simulink model "ExoskeletonControlModel"  (R2022b)
settings: Solver=ode3  StartTime=0.0  StopTime=inf  FixedStep=Ts  RelTol=1e-3
PreLoadFcn:
  | Ts_IO204 = 0.001;
  | 
  | if ~exist('Ts', 'var')
  | Ts = 0.001;
  | end
  | if ~exist('FPGA_Frequency', 'var')
  | FPGA_Frequency = 75000000;
  | end
  | 
  | ts_IO612 = 1e-3;
  | 
  | load('TargetReached.mat')
  | load('ActualPos_inc.mat')
model workspace (MAT data in the model file):
  DeltaData : timeseries (value not decoded)
  EC45_deg2incs = 2276
  EC60_deg2inc = 5461
  EC90_deg2incs = 7111
  Enc2rad_18bit = 2.3968e-05
  Enc2rad_19bit = 1.1984e-05
  Enc2rad_20bit = 5.9921e-06
  GiulioModel : robotics.RigidBodyTree (value not decoded)
  Giulio_Spheric_model : robotics.RigidBodyTree (value not decoded)
  Offset1_ticks = 571315
  Offset2_ticks = 590938.9928
  Offset3_ticks = 457912.8279
  Offset4_ticks = 482293.9763
  Offset5_ticks = 598735.9316
  Offset_M1 = 1.12645499896
  Offset_M2 = 4.02728553608
  Offset_M3 = 5.48587511336
  Offset_M4 = 2.03717511516
  Offset_M5 = 4.4996674016
  T1_Nm : object (value not decoded)
  T2_Nm : object (value not decoded)
  TBmodel : robotics.RigidBodyTree (value not decoded)
  Ts = 0.002
  Xg : object (value not decoded)
  Yg : object (value not decoded)
  Zg : object (value not decoded)
  a2 = 0.27
  change_variable = 0
  d1 = [0 0 0 0 0 0 0 0 0 0 0 0 ... (30001 elements, 30001x1)]
  d1_1 = 0.21074
  d2 = [0 0 0 0 0 0 0 0 0 0 0 0 ... (30001 elements, 30001x1)]
  d2_1 = 0.04864
  d3 = [0 0 0 0 0 0 0 0 0 0 0 0 ... (30001 elements, 30001x1)]
  d4 = [0 0 0 0 0 0 0 0 0 0 0 0 ... (30001 elements, 30001x1)]
  d5 = [0 0 0 0 0 0 0 0 0 0 0 0 ... (30001 elements, 30001x1)]
  d6 = [0 0 0 0 0 0 0 0 0 0 0 0 ... (30001 elements, 30001x1)]
  ee_x = -0.2852
  ee_y = -0.3683
  ee_z = -0.0386
  enc2rad_EC45 = 7.6699e-06
  enc2rad_EC90 = 2.3969e-05
  k1_Nm_ticks = 0.00923
  k2_Nm_ticks = 0.0257
  k3_Nm_ticks = 0.00692
  k4_Nm_ticks = 0.00729
  k5_Nm_ticks = 0.00641
  lower_lim_m1 = -330000
  lower_lim_m2 = -235302
  lower_lim_m3 = -132865
  lower_lim_m4 = -152732
  lower_lim_m5 = -138363
  lower_lim_m6 = -200325
  m1 = 2.441408578
  m2 = 3.750007
  m3 = 1.56250298
  m4 = 1.56250298
  m5 = 1.56250298
  m6 = 1.56250298
  n_oversampling = 8
  offset_sea_1 = 0.5547
  offset_sea_2 = 2.8595
  offset_sea_3 = 3.5058
  offset_sea_4 = 2.8586
  offset_sea_5 = 2.8736
  params : AKSIM (value not decoded)
  pos_th_neg = -180000
  pos_th_pos = 180000
  q1 = -1819347
  q2 = -196752
  q3 = -596465
  q4 = -556807
  q5 = -573932
  q6 = -489063
  sine = [0 0.187999937334 0.751998997352 1.69199492401 3.0079839574 4.6999608335 6.76791878442 9.21184953835 12.0317433196 15.2275888485 18.7993733417 22.7470825122 ... (12501 elements, 12501x1)]
  start : object (value not decoded)
  switch_admittance = 1
  t1 : object (value not decoded)
  t2 : object (value not decoded)
  torsionalStiffnes_M1 = 384.88
  torsionalStiffnes_M2 = 1500
  torsionalStiffnes_M3 = 901.97
  torsionalStiffnes_M4 = 950.86
  torsionalStiffnes_M5 = 930
  torsionalStiffnes_M6 = 914
  upper_lim_m1 = 340000
  upper_lim_m2 = 95467
  upper_lim_m3 = 164951
  upper_lim_m4 = 210607
  upper_lim_m5 = 252595
  upper_lim_m6 = 96694
  vel_th_neg = -100
  vel_th_pos = 100
  x = 0
undefined symbols (not defined in the file): C, DiscIntNeverNeededParam
libraries: canmsglib x285, speedgoatlib_IO614 x245, simulink x26, slrealtimeloglib x9, simulink_extras x6, robotmaniplib x6
(part 7 of 13)

== system ExoskeletonControlModel/DataProcessing/Working_Chart/GoHome.GoHome_M2.ST1_set_PPM_M2/receive_PDO2_m1 ==
  mode : Inport
  Bus Selector : BusSelector  OutputSignals=mode_m1,interpolation_period_m1
  CAN Write : speedgoatlib_IO614/CAN/CAN Write  id=1  sampleTime=-1  portSelection=3  messageType=CAN  enaStatusPort=off  protl=IO614  ptIdx=2  isFDMod=0
  set_mode : canmsglib/CAN Pack  MsgList=(none)  MsgName=CAN Msg  MsgIDType=Standard (11-bit identifier)  MsgIdentifier=hex2dec('302')  MsgLength=2  Remote=off  ApplyMinMax=off  BusOutput=off  SignalInfo={ 'mode', '0', '8', 'LE', 'unsigned', 'Standard', '0', '1', '0', '-Inf', 'Inf'; 'interpolation time period', '8', '8', 'LE', 'unsigned', 'Standard', '0', '1', '0', '-Inf', 'Inf' }
      settings: DataFormat=manually specified signals
  wires:
  set_mode/1 -> CAN Write/1
  mode/1 -> Bus Selector/1
  Bus Selector/1 -> set_mode/1  "<mode_m1>"
  Bus Selector/2 -> set_mode/2  "<interpolation_period_m1>"

== system ExoskeletonControlModel/DataProcessing/Working_Chart/GoHome.GoHome_M2.ST2_Switch_on_Enable_M2/receive_PDO1_m1 ==
  controlword : Inport
  CAN Write : speedgoatlib_IO614/CAN/CAN Write  id=1  sampleTime=-1  portSelection=3  messageType=CAN  enaStatusPort=off  protl=IO614  ptIdx=2  isFDMod=0
  set_controlword : canmsglib/CAN Pack  MsgList=(none)  MsgName=CAN Msg  MsgIDType=Standard (11-bit identifier)  MsgIdentifier=hex2dec('202')  MsgLength=2  Remote=off  ApplyMinMax=off  BusOutput=off  SignalInfo={ 'controlword', '0', '16', 'LE', 'unsigned', 'Standard', '0', '1', '0', '-Inf', 'Inf' }
      settings: DataFormat=manually specified signals
  wires:
  controlword/1 -> set_controlword/1
  set_controlword/1 -> CAN Write/1

== system ExoskeletonControlModel/DataProcessing/Working_Chart/GoHome.GoHome_M2.ST3_send_target_pos_M2/receive_PDO3_m1 ==
  target_pos : Inport
  CAN Write : speedgoatlib_IO614/CAN/CAN Write  id=1  sampleTime=-1  portSelection=3  messageType=CAN  enaStatusPort=off  protl=IO614  ptIdx=2  isFDMod=0
  set_position : canmsglib/CAN Pack  MsgList=(none)  MsgName=CAN Msg  MsgIDType=Standard (11-bit identifier)  MsgIdentifier=hex2dec('402')  MsgLength=4  Remote=off  ApplyMinMax=off  BusOutput=off  SignalInfo={ 'target position', '0', '32', 'LE', 'signed', 'Standard', '0', '1', '0', '-Inf', 'Inf' }
      settings: DataFormat=manually specified signals
  wires:
  target_pos/1 -> set_position/1
  set_position/1 -> CAN Write/1

== system ExoskeletonControlModel/DataProcessing/Working_Chart/GoHome.GoHome_M2.ST4_Abs_ref_start_immediatly_M2/receive_PDO1_m1 ==
  controlword : Inport
  CAN Write : speedgoatlib_IO614/CAN/CAN Write  id=1  sampleTime=-1  portSelection=3  messageType=CAN  enaStatusPort=off  protl=IO614  ptIdx=2  isFDMod=0
  set_controlword : canmsglib/CAN Pack  MsgList=(none)  MsgName=CAN Msg  MsgIDType=Standard (11-bit identifier)  MsgIdentifier=hex2dec('202')  MsgLength=2  Remote=off  ApplyMinMax=off  BusOutput=off  SignalInfo={ 'controlword', '0', '16', 'LE', 'unsigned', 'Standard', '0', '1', '0', '-Inf', 'Inf' }
      settings: DataFormat=manually specified signals
  wires:
  controlword/1 -> set_controlword/1
  set_controlword/1 -> CAN Write/1

== system ExoskeletonControlModel/DataProcessing/Working_Chart/GoHome.GoHome_M3.ST1_set_PPM_M3/receive_PDO2_m1 ==
  mode : Inport
  Bus Selector : BusSelector  OutputSignals=mode_m1,interpolation_period_m1
  CAN Write : speedgoatlib_IO614/CAN/CAN Write  id=1  sampleTime=-1  portSelection=4  messageType=CAN  enaStatusPort=off  protl=IO614  ptIdx=3  isFDMod=0
  set_mode : canmsglib/CAN Pack  MsgList=(none)  MsgName=CAN Msg  MsgIDType=Standard (11-bit identifier)  MsgIdentifier=hex2dec('301')  MsgLength=2  Remote=off  ApplyMinMax=off  BusOutput=off  SignalInfo={ 'mode', '0', '8', 'LE', 'unsigned', 'Standard', '0', '1', '0', '-Inf', 'Inf'; 'interpolation time period', '8', '8', 'LE', 'unsigned', 'Standard', '0', '1', '0', '-Inf', 'Inf' }
      settings: DataFormat=manually specified signals
  wires:
  set_mode/1 -> CAN Write/1
  mode/1 -> Bus Selector/1
  Bus Selector/1 -> set_mode/1  "<mode_m1>"
  Bus Selector/2 -> set_mode/2  "<interpolation_period_m1>"

== system ExoskeletonControlModel/DataProcessing/Working_Chart/GoHome.GoHome_M3.ST2_Switch_on_Enable_M3/receive_PDO1_m1 ==
  controlword : Inport
  CAN Write : speedgoatlib_IO614/CAN/CAN Write  id=1  sampleTime=-1  portSelection=4  messageType=CAN  enaStatusPort=off  protl=IO614  ptIdx=3  isFDMod=0
  set_controlword : canmsglib/CAN Pack  MsgList=(none)  MsgName=CAN Msg  MsgIDType=Standard (11-bit identifier)  MsgIdentifier=hex2dec('201')  MsgLength=2  Remote=off  ApplyMinMax=off  BusOutput=off  SignalInfo={ 'controlword', '0', '16', 'LE', 'unsigned', 'Standard', '0', '1', '0', '-Inf', 'Inf' }
      settings: DataFormat=manually specified signals
  wires:
  controlword/1 -> set_controlword/1
  set_controlword/1 -> CAN Write/1

== system ExoskeletonControlModel/DataProcessing/Working_Chart/GoHome.GoHome_M3.ST3_send_target_pos_M3/receive_PDO3_m1 ==
  target_pos : Inport
  CAN Write : speedgoatlib_IO614/CAN/CAN Write  id=1  sampleTime=-1  portSelection=4  messageType=CAN  enaStatusPort=off  protl=IO614  ptIdx=3  isFDMod=0
  set_position : canmsglib/CAN Pack  MsgList=(none)  MsgName=CAN Msg  MsgIDType=Standard (11-bit identifier)  MsgIdentifier=hex2dec('401')  MsgLength=4  Remote=off  ApplyMinMax=off  BusOutput=off  SignalInfo={ 'target position', '0', '32', 'LE', 'signed', 'Standard', '0', '1', '0', '-Inf', 'Inf' }
      settings: DataFormat=manually specified signals
  wires:
  target_pos/1 -> set_position/1
  set_position/1 -> CAN Write/1

== system ExoskeletonControlModel/DataProcessing/Working_Chart/GoHome.GoHome_M3.ST4_Abs_ref_start_immediatly_M3/receive_PDO1_m1 ==
  controlword : Inport
  CAN Write : speedgoatlib_IO614/CAN/CAN Write  id=1  sampleTime=-1  portSelection=4  messageType=CAN  enaStatusPort=off  protl=IO614  ptIdx=3  isFDMod=0
  set_controlword : canmsglib/CAN Pack  MsgList=(none)  MsgName=CAN Msg  MsgIDType=Standard (11-bit identifier)  MsgIdentifier=hex2dec('201')  MsgLength=2  Remote=off  ApplyMinMax=off  BusOutput=off  SignalInfo={ 'controlword', '0', '16', 'LE', 'unsigned', 'Standard', '0', '1', '0', '-Inf', 'Inf' }
      settings: DataFormat=manually specified signals
  wires:
  controlword/1 -> set_controlword/1
  set_controlword/1 -> CAN Write/1

== system ExoskeletonControlModel/DataProcessing/Working_Chart/GoHome.GoHome_M4.ST1_set_PPM_M4/receive_PDO2_m1 ==
  mode : Inport
  Bus Selector : BusSelector  OutputSignals=mode_m1,interpolation_period_m1
  CAN Write : speedgoatlib_IO614/CAN/CAN Write  id=1  sampleTime=-1  portSelection=4  messageType=CAN  enaStatusPort=off  protl=IO614  ptIdx=3  isFDMod=0
  set_mode : canmsglib/CAN Pack  MsgList=(none)  MsgName=CAN Msg  MsgIDType=Standard (11-bit identifier)  MsgIdentifier=hex2dec('302')  MsgLength=2  Remote=off  ApplyMinMax=off  BusOutput=off  SignalInfo={ 'mode', '0', '8', 'LE', 'unsigned', 'Standard', '0', '1', '0', '-Inf', 'Inf'; 'interpolation time period', '8', '8', 'LE', 'unsigned', 'Standard', '0', '1', '0', '-Inf', 'Inf' }
      settings: DataFormat=manually specified signals
  wires:
  set_mode/1 -> CAN Write/1
  mode/1 -> Bus Selector/1
  Bus Selector/1 -> set_mode/1  "<mode_m1>"
  Bus Selector/2 -> set_mode/2  "<interpolation_period_m1>"

== system ExoskeletonControlModel/DataProcessing/Working_Chart/GoHome.GoHome_M4.ST2_Switch_on_Enable_M4/receive_PDO1_m1 ==
  controlword : Inport
  CAN Write : speedgoatlib_IO614/CAN/CAN Write  id=1  sampleTime=-1  portSelection=4  messageType=CAN  enaStatusPort=off  protl=IO614  ptIdx=3  isFDMod=0
  set_controlword : canmsglib/CAN Pack  MsgList=(none)  MsgName=CAN Msg  MsgIDType=Standard (11-bit identifier)  MsgIdentifier=hex2dec('202')  MsgLength=2  Remote=off  ApplyMinMax=off  BusOutput=off  SignalInfo={ 'controlword', '0', '16', 'LE', 'unsigned', 'Standard', '0', '1', '0', '-Inf', 'Inf' }
      settings: DataFormat=manually specified signals
  wires:
  controlword/1 -> set_controlword/1
  set_controlword/1 -> CAN Write/1

== system ExoskeletonControlModel/DataProcessing/Working_Chart/GoHome.GoHome_M4.ST3_send_target_pos_M4/receive_PDO3_m1 ==
  target_pos : Inport
  CAN Write : speedgoatlib_IO614/CAN/CAN Write  id=1  sampleTime=-1  portSelection=4  messageType=CAN  enaStatusPort=off  protl=IO614  ptIdx=3  isFDMod=0
  set_position : canmsglib/CAN Pack  MsgList=(none)  MsgName=CAN Msg  MsgIDType=Standard (11-bit identifier)  MsgIdentifier=hex2dec('402')  MsgLength=4  Remote=off  ApplyMinMax=off  BusOutput=off  SignalInfo={ 'target position', '0', '32', 'LE', 'signed', 'Standard', '0', '1', '0', '-Inf', 'Inf' }
      settings: DataFormat=manually specified signals
  wires:
  target_pos/1 -> set_position/1
  set_position/1 -> CAN Write/1

== system ExoskeletonControlModel/DataProcessing/Working_Chart/GoHome.GoHome_M4.ST4_Abs_ref_start_immediatly_M4/receive_PDO1_m1 ==
  controlword : Inport
  CAN Write : speedgoatlib_IO614/CAN/CAN Write  id=1  sampleTime=-1  portSelection=4  messageType=CAN  enaStatusPort=off  protl=IO614  ptIdx=3  isFDMod=0
  set_controlword : canmsglib/CAN Pack  MsgList=(none)  MsgName=CAN Msg  MsgIDType=Standard (11-bit identifier)  MsgIdentifier=hex2dec('202')  MsgLength=2  Remote=off  ApplyMinMax=off  BusOutput=off  SignalInfo={ 'controlword', '0', '16', 'LE', 'unsigned', 'Standard', '0', '1', '0', '-Inf', 'Inf' }
      settings: DataFormat=manually specified signals
  wires:
  controlword/1 -> set_controlword/1
  set_controlword/1 -> CAN Write/1

== system ExoskeletonControlModel/DataProcessing/Working_Chart/GoHome.GoHome_M5.ST1_set_PPM_M5/receive_PDO2_m1 ==
  mode : Inport
  Bus Selector : BusSelector  OutputSignals=mode_m1,interpolation_period_m1
  CAN Write : speedgoatlib_IO614/CAN/CAN Write  id=1  sampleTime=-1  portSelection=4  messageType=CAN  enaStatusPort=off  protl=IO614  ptIdx=3  isFDMod=0
  set_mode : canmsglib/CAN Pack  MsgList=(none)  MsgName=CAN Msg  MsgIDType=Standard (11-bit identifier)  MsgIdentifier=hex2dec('303')  MsgLength=2  Remote=off  ApplyMinMax=off  BusOutput=off  SignalInfo={ 'mode', '0', '8', 'LE', 'unsigned', 'Standard', '0', '1', '0', '-Inf', 'Inf'; 'interpolation time period', '8', '8', 'LE', 'unsigned', 'Standard', '0', '1', '0', '-Inf', 'Inf' }
      settings: DataFormat=manually specified signals
  wires:
  set_mode/1 -> CAN Write/1
  mode/1 -> Bus Selector/1
  Bus Selector/1 -> set_mode/1  "<mode_m1>"
  Bus Selector/2 -> set_mode/2  "<interpolation_period_m1>"

== system ExoskeletonControlModel/DataProcessing/Working_Chart/GoHome.GoHome_M5.ST2_Switch_on_Enable_M5/receive_PDO1_m1 ==
  controlword : Inport
  CAN Write : speedgoatlib_IO614/CAN/CAN Write  id=1  sampleTime=-1  portSelection=4  messageType=CAN  enaStatusPort=off  protl=IO614  ptIdx=3  isFDMod=0
  set_controlword : canmsglib/CAN Pack  MsgList=(none)  MsgName=CAN Msg  MsgIDType=Standard (11-bit identifier)  MsgIdentifier=hex2dec('203')  MsgLength=2  Remote=off  ApplyMinMax=off  BusOutput=off  SignalInfo={ 'controlword', '0', '16', 'LE', 'unsigned', 'Standard', '0', '1', '0', '-Inf', 'Inf' }
      settings: DataFormat=manually specified signals
  wires:
  controlword/1 -> set_controlword/1
  set_controlword/1 -> CAN Write/1

== system ExoskeletonControlModel/DataProcessing/Working_Chart/GoHome.GoHome_M5.ST3_send_target_pos_M5/receive_PDO3_m1 ==
  target_pos : Inport
  CAN Write : speedgoatlib_IO614/CAN/CAN Write  id=1  sampleTime=-1  portSelection=4  messageType=CAN  enaStatusPort=off  protl=IO614  ptIdx=3  isFDMod=0
  set_position : canmsglib/CAN Pack  MsgList=(none)  MsgName=CAN Msg  MsgIDType=Standard (11-bit identifier)  MsgIdentifier=hex2dec('403')  MsgLength=4  Remote=off  ApplyMinMax=off  BusOutput=off  SignalInfo={ 'target position', '0', '32', 'LE', 'signed', 'Standard', '0', '1', '0', '-Inf', 'Inf' }
      settings: DataFormat=manually specified signals
  wires:
  target_pos/1 -> set_position/1
  set_position/1 -> CAN Write/1

== system ExoskeletonControlModel/DataProcessing/Working_Chart/GoHome.GoHome_M5.ST4_Abs_ref_start_immediatly_M5/receive_PDO1_m1 ==
  controlword : Inport
  CAN Write : speedgoatlib_IO614/CAN/CAN Write  id=1  sampleTime=-1  portSelection=4  messageType=CAN  enaStatusPort=off  protl=IO614  ptIdx=3  isFDMod=0
  set_controlword : canmsglib/CAN Pack  MsgList=(none)  MsgName=CAN Msg  MsgIDType=Standard (11-bit identifier)  MsgIdentifier=hex2dec('203')  MsgLength=2  Remote=off  ApplyMinMax=off  BusOutput=off  SignalInfo={ 'controlword', '0', '16', 'LE', 'unsigned', 'Standard', '0', '1', '0', '-Inf', 'Inf' }
      settings: DataFormat=manually specified signals
  wires:
  controlword/1 -> set_controlword/1
  set_controlword/1 -> CAN Write/1

== system ExoskeletonControlModel/DataProcessing/Working_Chart/GoHome.GoHome_M6.ST1_set_PPM_M6/receive_PDO2_m1 ==
  mode : Inport
  Bus Selector : BusSelector  OutputSignals=mode_m1,interpolation_period_m1
  CAN Write : speedgoatlib_IO614/CAN/CAN Write  id=1  sampleTime=-1  portSelection=4  messageType=CAN  enaStatusPort=off  protl=IO614  ptIdx=3  isFDMod=0
  set_mode : canmsglib/CAN Pack  MsgList=(none)  MsgName=CAN Msg  MsgIDType=Standard (11-bit identifier)  MsgIdentifier=hex2dec('304')  MsgLength=2  Remote=off  ApplyMinMax=off  BusOutput=off  SignalInfo={ 'mode', '0', '8', 'LE', 'unsigned', 'Standard', '0', '1', '0', '-Inf', 'Inf'; 'interpolation time period', '8', '8', 'LE', 'unsigned', 'Standard', '0', '1', '0', '-Inf', 'Inf' }
      settings: DataFormat=manually specified signals
  wires:
  set_mode/1 -> CAN Write/1
  mode/1 -> Bus Selector/1
  Bus Selector/1 -> set_mode/1  "<mode_m1>"
  Bus Selector/2 -> set_mode/2  "<interpolation_period_m1>"

== system ExoskeletonControlModel/DataProcessing/Working_Chart/GoHome.GoHome_M6.ST2_Switch_on_Enable_M6/receive_PDO1_m1 ==
  controlword : Inport
  CAN Write : speedgoatlib_IO614/CAN/CAN Write  id=1  sampleTime=-1  portSelection=4  messageType=CAN  enaStatusPort=off  protl=IO614  ptIdx=3  isFDMod=0
  set_controlword : canmsglib/CAN Pack  MsgList=(none)  MsgName=CAN Msg  MsgIDType=Standard (11-bit identifier)  MsgIdentifier=hex2dec('204')  MsgLength=2  Remote=off  ApplyMinMax=off  BusOutput=off  SignalInfo={ 'controlword', '0', '16', 'LE', 'unsigned', 'Standard', '0', '1', '0', '-Inf', 'Inf' }
      settings: DataFormat=manually specified signals
  wires:
  controlword/1 -> set_controlword/1
  set_controlword/1 -> CAN Write/1

== system ExoskeletonControlModel/DataProcessing/Working_Chart/GoHome.GoHome_M6.ST3_send_target_pos_M6/receive_PDO3_m1 ==
  target_pos : Inport
  CAN Write : speedgoatlib_IO614/CAN/CAN Write  id=1  sampleTime=-1  portSelection=4  messageType=CAN  enaStatusPort=off  protl=IO614  ptIdx=3  isFDMod=0
  set_position : canmsglib/CAN Pack  MsgList=(none)  MsgName=CAN Msg  MsgIDType=Standard (11-bit identifier)  MsgIdentifier=hex2dec('404')  MsgLength=4  Remote=off  ApplyMinMax=off  BusOutput=off  SignalInfo={ 'target position', '0', '32', 'LE', 'signed', 'Standard', '0', '1', '0', '-Inf', 'Inf' }
      settings: DataFormat=manually specified signals
  wires:
  target_pos/1 -> set_position/1
  set_position/1 -> CAN Write/1

== system ExoskeletonControlModel/DataProcessing/Working_Chart/GoHome.GoHome_M6.ST4_Abs_ref_start_immediatly_M6/receive_PDO1_m1 ==
  controlword : Inport
  CAN Write : speedgoatlib_IO614/CAN/CAN Write  id=1  sampleTime=-1  portSelection=4  messageType=CAN  enaStatusPort=off  protl=IO614  ptIdx=3  isFDMod=0
  set_controlword : canmsglib/CAN Pack  MsgList=(none)  MsgName=CAN Msg  MsgIDType=Standard (11-bit identifier)  MsgIdentifier=hex2dec('204')  MsgLength=2  Remote=off  ApplyMinMax=off  BusOutput=off  SignalInfo={ 'controlword', '0', '16', 'LE', 'unsigned', 'Standard', '0', '1', '0', '-Inf', 'Inf' }
      settings: DataFormat=manually specified signals
  wires:
  controlword/1 -> set_controlword/1
  set_controlword/1 -> CAN Write/1

== system ExoskeletonControlModel/DataProcessing/Working_Chart/Transparency.Block_not_recorded_joints.ST1_set_CSP_M1/receive_PDO2_m1 ==
  mode : Inport
  Bus Selector : BusSelector  OutputSignals=mode_m1,interpolation_period_m1
  CAN Write : speedgoatlib_IO614/CAN/CAN Write  id=1  sampleTime=-1  portSelection=3  messageType=CAN  enaStatusPort=off  protl=IO614  ptIdx=2  isFDMod=0
  set_mode : canmsglib/CAN Pack  MsgList=(none)  MsgName=CAN Msg  MsgIDType=Standard (11-bit identifier)  MsgIdentifier=hex2dec('301')  MsgLength=2  Remote=off  ApplyMinMax=off  BusOutput=off  SignalInfo={ 'mode', '0', '8', 'LE', 'unsigned', 'Standard', '0', '1', '0', '-Inf', 'Inf'; 'interpolation time period', '8', '8', 'LE', 'unsigned', 'Standard', '0', '1', '0', '-Inf', 'Inf' }
      settings: DataFormat=manually specified signals
  wires:
  set_mode/1 -> CAN Write/1
  mode/1 -> Bus Selector/1
  Bus Selector/1 -> set_mode/1  "<mode_m1>"
  Bus Selector/2 -> set_mode/2  "<interpolation_period_m1>"

== system ExoskeletonControlModel/DataProcessing/Working_Chart/Transparency.Block_not_recorded_joints.ST1_set_CSP_M6/receive_PDO2_m1 ==
  mode : Inport
  Bus Selector : BusSelector  OutputSignals=mode_m1,interpolation_period_m1
  CAN Write : speedgoatlib_IO614/CAN/CAN Write  id=1  sampleTime=-1  portSelection=4  messageType=CAN  enaStatusPort=off  protl=IO614  ptIdx=3  isFDMod=0
  set_mode : canmsglib/CAN Pack  MsgList=(none)  MsgName=CAN Msg  MsgIDType=Standard (11-bit identifier)  MsgIdentifier=hex2dec('304')  MsgLength=2  Remote=off  ApplyMinMax=off  BusOutput=off  SignalInfo={ 'mode', '0', '8', 'LE', 'unsigned', 'Standard', '0', '1', '0', '-Inf', 'Inf'; 'interpolation time period', '8', '8', 'LE', 'unsigned', 'Standard', '0', '1', '0', '-Inf', 'Inf' }
      settings: DataFormat=manually specified signals
  wires:
  set_mode/1 -> CAN Write/1
  mode/1 -> Bus Selector/1
  Bus Selector/1 -> set_mode/1  "<mode_m1>"
  Bus Selector/2 -> set_mode/2  "<interpolation_period_m1>"

== system ExoskeletonControlModel/DataProcessing/Working_Chart/Transparency.GoToExerciseHome.GoHome_M1.ST1_set_PPM_M1/receive_PDO2_m1 ==
  mode : Inport
  Bus Selector : BusSelector  OutputSignals=mode_m1,interpolation_period_m1
  CAN Write : speedgoatlib_IO614/CAN/CAN Write  id=1  sampleTime=-1  portSelection=3  messageType=CAN  enaStatusPort=off  protl=IO614  ptIdx=2  isFDMod=0
  set_mode : canmsglib/CAN Pack  MsgList=(none)  MsgName=CAN Msg  MsgIDType=Standard (11-bit identifier)  MsgIdentifier=hex2dec('301')  MsgLength=2  Remote=off  ApplyMinMax=off  BusOutput=off  SignalInfo={ 'mode', '0', '8', 'LE', 'unsigned', 'Standard', '0', '1', '0', '-Inf', 'Inf'; 'interpolation time period', '8', '8', 'LE', 'unsigned', 'Standard', '0', '1', '0', '-Inf', 'Inf' }
      settings: DataFormat=manually specified signals
  wires:
  set_mode/1 -> CAN Write/1
  mode/1 -> Bus Selector/1
  Bus Selector/1 -> set_mode/1  "<mode_m1>"
  Bus Selector/2 -> set_mode/2  "<interpolation_period_m1>"

== system ExoskeletonControlModel/DataProcessing/Working_Chart/Transparency.GoToExerciseHome.GoHome_M1.ST2_Switch_on_Enable_M1/receive_PDO1_m1 ==
  controlword : Inport
  CAN Write : speedgoatlib_IO614/CAN/CAN Write  id=1  sampleTime=-1  portSelection=3  messageType=CAN  enaStatusPort=off  protl=IO614  ptIdx=2  isFDMod=0
  set_controlword : canmsglib/CAN Pack  MsgList=(none)  MsgName=CAN Msg  MsgIDType=Standard (11-bit identifier)  MsgIdentifier=hex2dec('201')  MsgLength=2  Remote=off  ApplyMinMax=off  BusOutput=off  SignalInfo={ 'controlword', '0', '16', 'LE', 'unsigned', 'Standard', '0', '1', '0', '-Inf', 'Inf' }
      settings: DataFormat=manually specified signals
  wires:
  controlword/1 -> set_controlword/1
  set_controlword/1 -> CAN Write/1

== system ExoskeletonControlModel/DataProcessing/Working_Chart/Transparency.GoToExerciseHome.GoHome_M1.ST3_send_target_pos_M1/receive_PDO3_m1 ==
  target_pos : Inport
  CAN Write : speedgoatlib_IO614/CAN/CAN Write  id=1  sampleTime=-1  portSelection=3  messageType=CAN  enaStatusPort=off  protl=IO614  ptIdx=2  isFDMod=0
  set_position : canmsglib/CAN Pack  MsgList=(none)  MsgName=CAN Msg  MsgIDType=Standard (11-bit identifier)  MsgIdentifier=hex2dec('401')  MsgLength=4  Remote=off  ApplyMinMax=off  BusOutput=off  SignalInfo={ 'target position', '0', '32', 'LE', 'signed', 'Standard', '0', '1', '0', '-Inf', 'Inf' }
      settings: DataFormat=manually specified signals
  wires:
  target_pos/1 -> set_position/1
  set_position/1 -> CAN Write/1

== system ExoskeletonControlModel/DataProcessing/Working_Chart/Transparency.GoToExerciseHome.GoHome_M1.ST4_Abs_ref_start_immediatly_M1/receive_PDO1_m1 ==
  controlword : Inport
  CAN Write : speedgoatlib_IO614/CAN/CAN Write  id=1  sampleTime=-1  portSelection=3  messageType=CAN  enaStatusPort=off  protl=IO614  ptIdx=2  isFDMod=0
  set_controlword : canmsglib/CAN Pack  MsgList=(none)  MsgName=CAN Msg  MsgIDType=Standard (11-bit identifier)  MsgIdentifier=hex2dec('201')  MsgLength=2  Remote=off  ApplyMinMax=off  BusOutput=off  SignalInfo={ 'controlword', '0', '16', 'LE', 'unsigned', 'Standard', '0', '1', '0', '-Inf', 'Inf' }
      settings: DataFormat=manually specified signals
  wires:
  controlword/1 -> set_controlword/1
  set_controlword/1 -> CAN Write/1

== system ExoskeletonControlModel/DataProcessing/Working_Chart/Transparency.GoToExerciseHome.GoHome_M2.ST1_set_PPM_M2/receive_PDO2_m1 ==
  mode : Inport
  Bus Selector : BusSelector  OutputSignals=mode_m1,interpolation_period_m1
  CAN Write : speedgoatlib_IO614/CAN/CAN Write  id=1  sampleTime=-1  portSelection=3  messageType=CAN  enaStatusPort=off  protl=IO614  ptIdx=2  isFDMod=0
  set_mode : canmsglib/CAN Pack  MsgList=(none)  MsgName=CAN Msg  MsgIDType=Standard (11-bit identifier)  MsgIdentifier=hex2dec('302')  MsgLength=2  Remote=off  ApplyMinMax=off  BusOutput=off  SignalInfo={ 'mode', '0', '8', 'LE', 'unsigned', 'Standard', '0', '1', '0', '-Inf', 'Inf'; 'interpolation time period', '8', '8', 'LE', 'unsigned', 'Standard', '0', '1', '0', '-Inf', 'Inf' }
      settings: DataFormat=manually specified signals
  wires:
  set_mode/1 -> CAN Write/1
  mode/1 -> Bus Selector/1
  Bus Selector/1 -> set_mode/1  "<mode_m1>"
  Bus Selector/2 -> set_mode/2  "<interpolation_period_m1>"

== system ExoskeletonControlModel/DataProcessing/Working_Chart/Transparency.GoToExerciseHome.GoHome_M2.ST2_Switch_on_Enable_M2/receive_PDO1_m1 ==
  controlword : Inport
  CAN Write : speedgoatlib_IO614/CAN/CAN Write  id=1  sampleTime=-1  portSelection=3  messageType=CAN  enaStatusPort=off  protl=IO614  ptIdx=2  isFDMod=0
  set_controlword : canmsglib/CAN Pack  MsgList=(none)  MsgName=CAN Msg  MsgIDType=Standard (11-bit identifier)  MsgIdentifier=hex2dec('202')  MsgLength=2  Remote=off  ApplyMinMax=off  BusOutput=off  SignalInfo={ 'controlword', '0', '16', 'LE', 'unsigned', 'Standard', '0', '1', '0', '-Inf', 'Inf' }
      settings: DataFormat=manually specified signals
  wires:
  controlword/1 -> set_controlword/1
  set_controlword/1 -> CAN Write/1

== system ExoskeletonControlModel/DataProcessing/Working_Chart/Transparency.GoToExerciseHome.GoHome_M2.ST3_send_target_pos_M2/receive_PDO3_m1 ==
  target_pos : Inport
  CAN Write : speedgoatlib_IO614/CAN/CAN Write  id=1  sampleTime=-1  portSelection=3  messageType=CAN  enaStatusPort=off  protl=IO614  ptIdx=2  isFDMod=0
  set_position : canmsglib/CAN Pack  MsgList=(none)  MsgName=CAN Msg  MsgIDType=Standard (11-bit identifier)  MsgIdentifier=hex2dec('402')  MsgLength=4  Remote=off  ApplyMinMax=off  BusOutput=off  SignalInfo={ 'target position', '0', '32', 'LE', 'signed', 'Standard', '0', '1', '0', '-Inf', 'Inf' }
      settings: DataFormat=manually specified signals
  wires:
  target_pos/1 -> set_position/1
  set_position/1 -> CAN Write/1

== system ExoskeletonControlModel/DataProcessing/Working_Chart/Transparency.GoToExerciseHome.GoHome_M2.ST4_Abs_ref_start_immediatly_M2/receive_PDO1_m1 ==
  controlword : Inport
  CAN Write : speedgoatlib_IO614/CAN/CAN Write  id=1  sampleTime=-1  portSelection=3  messageType=CAN  enaStatusPort=off  protl=IO614  ptIdx=2  isFDMod=0
  set_controlword : canmsglib/CAN Pack  MsgList=(none)  MsgName=CAN Msg  MsgIDType=Standard (11-bit identifier)  MsgIdentifier=hex2dec('202')  MsgLength=2  Remote=off  ApplyMinMax=off  BusOutput=off  SignalInfo={ 'controlword', '0', '16', 'LE', 'unsigned', 'Standard', '0', '1', '0', '-Inf', 'Inf' }
      settings: DataFormat=manually specified signals
  wires:
  controlword/1 -> set_controlword/1
  set_controlword/1 -> CAN Write/1

== system ExoskeletonControlModel/DataProcessing/Working_Chart/Transparency.GoToExerciseHome.GoHome_M3.ST1_set_PPM_M3/receive_PDO2_m1 ==
  mode : Inport
  Bus Selector : BusSelector  OutputSignals=mode_m1,interpolation_period_m1
  CAN Write : speedgoatlib_IO614/CAN/CAN Write  id=1  sampleTime=-1  portSelection=4  messageType=CAN  enaStatusPort=off  protl=IO614  ptIdx=3  isFDMod=0
  set_mode : canmsglib/CAN Pack  MsgList=(none)  MsgName=CAN Msg  MsgIDType=Standard (11-bit identifier)  MsgIdentifier=hex2dec('301')  MsgLength=2  Remote=off  ApplyMinMax=off  BusOutput=off  SignalInfo={ 'mode', '0', '8', 'LE', 'unsigned', 'Standard', '0', '1', '0', '-Inf', 'Inf'; 'interpolation time period', '8', '8', 'LE', 'unsigned', 'Standard', '0', '1', '0', '-Inf', 'Inf' }
      settings: DataFormat=manually specified signals
  wires:
  set_mode/1 -> CAN Write/1
  mode/1 -> Bus Selector/1
  Bus Selector/1 -> set_mode/1  "<mode_m1>"
  Bus Selector/2 -> set_mode/2  "<interpolation_period_m1>"

== system ExoskeletonControlModel/DataProcessing/Working_Chart/Transparency.GoToExerciseHome.GoHome_M3.ST2_Switch_on_Enable_M3/receive_PDO1_m1 ==
  controlword : Inport
  CAN Write : speedgoatlib_IO614/CAN/CAN Write  id=1  sampleTime=-1  portSelection=4  messageType=CAN  enaStatusPort=off  protl=IO614  ptIdx=3  isFDMod=0
  set_controlword : canmsglib/CAN Pack  MsgList=(none)  MsgName=CAN Msg  MsgIDType=Standard (11-bit identifier)  MsgIdentifier=hex2dec('201')  MsgLength=2  Remote=off  ApplyMinMax=off  BusOutput=off  SignalInfo={ 'controlword', '0', '16', 'LE', 'unsigned', 'Standard', '0', '1', '0', '-Inf', 'Inf' }
      settings: DataFormat=manually specified signals
  wires:
  controlword/1 -> set_controlword/1
  set_controlword/1 -> CAN Write/1

== system ExoskeletonControlModel/DataProcessing/Working_Chart/Transparency.GoToExerciseHome.GoHome_M3.ST3_send_target_pos_M3/receive_PDO3_m1 ==
  target_pos : Inport
  CAN Write : speedgoatlib_IO614/CAN/CAN Write  id=1  sampleTime=-1  portSelection=4  messageType=CAN  enaStatusPort=off  protl=IO614  ptIdx=3  isFDMod=0
  set_position : canmsglib/CAN Pack  MsgList=(none)  MsgName=CAN Msg  MsgIDType=Standard (11-bit identifier)  MsgIdentifier=hex2dec('401')  MsgLength=4  Remote=off  ApplyMinMax=off  BusOutput=off  SignalInfo={ 'target position', '0', '32', 'LE', 'signed', 'Standard', '0', '1', '0', '-Inf', 'Inf' }
      settings: DataFormat=manually specified signals
  wires:
  target_pos/1 -> set_position/1
  set_position/1 -> CAN Write/1

== system ExoskeletonControlModel/DataProcessing/Working_Chart/Transparency.GoToExerciseHome.GoHome_M3.ST4_Abs_ref_start_immediatly_M3/receive_PDO1_m1 ==
  controlword : Inport
  CAN Write : speedgoatlib_IO614/CAN/CAN Write  id=1  sampleTime=-1  portSelection=4  messageType=CAN  enaStatusPort=off  protl=IO614  ptIdx=3  isFDMod=0
  set_controlword : canmsglib/CAN Pack  MsgList=(none)  MsgName=CAN Msg  MsgIDType=Standard (11-bit identifier)  MsgIdentifier=hex2dec('201')  MsgLength=2  Remote=off  ApplyMinMax=off  BusOutput=off  SignalInfo={ 'controlword', '0', '16', 'LE', 'unsigned', 'Standard', '0', '1', '0', '-Inf', 'Inf' }
      settings: DataFormat=manually specified signals
  wires:
  controlword/1 -> set_controlword/1
  set_controlword/1 -> CAN Write/1

== system ExoskeletonControlModel/DataProcessing/Working_Chart/Transparency.GoToExerciseHome.GoHome_M4.ST1_set_PPM_M4/receive_PDO2_m1 ==
  mode : Inport
  Bus Selector : BusSelector  OutputSignals=mode_m1,interpolation_period_m1
  CAN Write : speedgoatlib_IO614/CAN/CAN Write  id=1  sampleTime=-1  portSelection=4  messageType=CAN  enaStatusPort=off  protl=IO614  ptIdx=3  isFDMod=0
  set_mode : canmsglib/CAN Pack  MsgList=(none)  MsgName=CAN Msg  MsgIDType=Standard (11-bit identifier)  MsgIdentifier=hex2dec('302')  MsgLength=2  Remote=off  ApplyMinMax=off  BusOutput=off  SignalInfo={ 'mode', '0', '8', 'LE', 'unsigned', 'Standard', '0', '1', '0', '-Inf', 'Inf'; 'interpolation time period', '8', '8', 'LE', 'unsigned', 'Standard', '0', '1', '0', '-Inf', 'Inf' }
      settings: DataFormat=manually specified signals
  wires:
  set_mode/1 -> CAN Write/1
  mode/1 -> Bus Selector/1
  Bus Selector/1 -> set_mode/1  "<mode_m1>"
  Bus Selector/2 -> set_mode/2  "<interpolation_period_m1>"

== system ExoskeletonControlModel/DataProcessing/Working_Chart/Transparency.GoToExerciseHome.GoHome_M4.ST2_Switch_on_Enable_M4/receive_PDO1_m1 ==
  controlword : Inport
  CAN Write : speedgoatlib_IO614/CAN/CAN Write  id=1  sampleTime=-1  portSelection=4  messageType=CAN  enaStatusPort=off  protl=IO614  ptIdx=3  isFDMod=0
  set_controlword : canmsglib/CAN Pack  MsgList=(none)  MsgName=CAN Msg  MsgIDType=Standard (11-bit identifier)  MsgIdentifier=hex2dec('202')  MsgLength=2  Remote=off  ApplyMinMax=off  BusOutput=off  SignalInfo={ 'controlword', '0', '16', 'LE', 'unsigned', 'Standard', '0', '1', '0', '-Inf', 'Inf' }
      settings: DataFormat=manually specified signals
  wires:
  controlword/1 -> set_controlword/1
  set_controlword/1 -> CAN Write/1

== system ExoskeletonControlModel/DataProcessing/Working_Chart/Transparency.GoToExerciseHome.GoHome_M4.ST3_send_target_pos_M4/receive_PDO3_m1 ==
  target_pos : Inport
  CAN Write : speedgoatlib_IO614/CAN/CAN Write  id=1  sampleTime=-1  portSelection=4  messageType=CAN  enaStatusPort=off  protl=IO614  ptIdx=3  isFDMod=0
  set_position : canmsglib/CAN Pack  MsgList=(none)  MsgName=CAN Msg  MsgIDType=Standard (11-bit identifier)  MsgIdentifier=hex2dec('402')  MsgLength=4  Remote=off  ApplyMinMax=off  BusOutput=off  SignalInfo={ 'target position', '0', '32', 'LE', 'signed', 'Standard', '0', '1', '0', '-Inf', 'Inf' }
      settings: DataFormat=manually specified signals
  wires:
  target_pos/1 -> set_position/1
  set_position/1 -> CAN Write/1

== system ExoskeletonControlModel/DataProcessing/Working_Chart/Transparency.GoToExerciseHome.GoHome_M4.ST3_send_target_pos_M4_abd/receive_PDO3_m1 ==
  target_pos : Inport
  CAN Write : speedgoatlib_IO614/CAN/CAN Write  id=1  sampleTime=-1  portSelection=4  messageType=CAN  enaStatusPort=off  protl=IO614  ptIdx=3  isFDMod=0
  set_position : canmsglib/CAN Pack  MsgList=(none)  MsgName=CAN Msg  MsgIDType=Standard (11-bit identifier)  MsgIdentifier=hex2dec('402')  MsgLength=4  Remote=off  ApplyMinMax=off  BusOutput=off  SignalInfo={ 'target position', '0', '32', 'LE', 'signed', 'Standard', '0', '1', '0', '-Inf', 'Inf' }
      settings: DataFormat=manually specified signals
  wires:
  target_pos/1 -> set_position/1
  set_position/1 -> CAN Write/1

== system ExoskeletonControlModel/DataProcessing/Working_Chart/Transparency.GoToExerciseHome.GoHome_M4.ST4_Abs_ref_start_immediatly_M4/receive_PDO1_m1 ==
  controlword : Inport
  CAN Write : speedgoatlib_IO614/CAN/CAN Write  id=1  sampleTime=-1  portSelection=4  messageType=CAN  enaStatusPort=off  protl=IO614  ptIdx=3  isFDMod=0
  set_controlword : canmsglib/CAN Pack  MsgList=(none)  MsgName=CAN Msg  MsgIDType=Standard (11-bit identifier)  MsgIdentifier=hex2dec('202')  MsgLength=2  Remote=off  ApplyMinMax=off  BusOutput=off  SignalInfo={ 'controlword', '0', '16', 'LE', 'unsigned', 'Standard', '0', '1', '0', '-Inf', 'Inf' }
      settings: DataFormat=manually specified signals
  wires:
  controlword/1 -> set_controlword/1
  set_controlword/1 -> CAN Write/1

== system ExoskeletonControlModel/DataProcessing/Working_Chart/Transparency.GoToExerciseHome.GoHome_M5.ST1_set_PPM_M5/receive_PDO2_m1 ==
  mode : Inport
  Bus Selector : BusSelector  OutputSignals=mode_m1,interpolation_period_m1
  CAN Write : speedgoatlib_IO614/CAN/CAN Write  id=1  sampleTime=-1  portSelection=4  messageType=CAN  enaStatusPort=off  protl=IO614  ptIdx=3  isFDMod=0
  set_mode : canmsglib/CAN Pack  MsgList=(none)  MsgName=CAN Msg  MsgIDType=Standard (11-bit identifier)  MsgIdentifier=hex2dec('303')  MsgLength=2  Remote=off  ApplyMinMax=off  BusOutput=off  SignalInfo={ 'mode', '0', '8', 'LE', 'unsigned', 'Standard', '0', '1', '0', '-Inf', 'Inf'; 'interpolation time period', '8', '8', 'LE', 'unsigned', 'Standard', '0', '1', '0', '-Inf', 'Inf' }
      settings: DataFormat=manually specified signals
  wires:
  set_mode/1 -> CAN Write/1
  mode/1 -> Bus Selector/1
  Bus Selector/1 -> set_mode/1  "<mode_m1>"
  Bus Selector/2 -> set_mode/2  "<interpolation_period_m1>"

== system ExoskeletonControlModel/DataProcessing/Working_Chart/Transparency.GoToExerciseHome.GoHome_M5.ST2_Switch_on_Enable_M5/receive_PDO1_m1 ==
  controlword : Inport
  CAN Write : speedgoatlib_IO614/CAN/CAN Write  id=1  sampleTime=-1  portSelection=4  messageType=CAN  enaStatusPort=off  protl=IO614  ptIdx=3  isFDMod=0
  set_controlword : canmsglib/CAN Pack  MsgList=(none)  MsgName=CAN Msg  MsgIDType=Standard (11-bit identifier)  MsgIdentifier=hex2dec('203')  MsgLength=2  Remote=off  ApplyMinMax=off  BusOutput=off  SignalInfo={ 'controlword', '0', '16', 'LE', 'unsigned', 'Standard', '0', '1', '0', '-Inf', 'Inf' }
      settings: DataFormat=manually specified signals
  wires:
  controlword/1 -> set_controlword/1
  set_controlword/1 -> CAN Write/1

== system ExoskeletonControlModel/DataProcessing/Working_Chart/Transparency.GoToExerciseHome.GoHome_M5.ST3_send_target_pos_M5/receive_PDO3_m1 ==
  target_pos : Inport
  CAN Write : speedgoatlib_IO614/CAN/CAN Write  id=1  sampleTime=-1  portSelection=4  messageType=CAN  enaStatusPort=off  protl=IO614  ptIdx=3  isFDMod=0
  set_position : canmsglib/CAN Pack  MsgList=(none)  MsgName=CAN Msg  MsgIDType=Standard (11-bit identifier)  MsgIdentifier=hex2dec('403')  MsgLength=4  Remote=off  ApplyMinMax=off  BusOutput=off  SignalInfo={ 'target position', '0', '32', 'LE', 'signed', 'Standard', '0', '1', '0', '-Inf', 'Inf' }
      settings: DataFormat=manually specified signals
  wires:
  target_pos/1 -> set_position/1
  set_position/1 -> CAN Write/1

== system ExoskeletonControlModel/DataProcessing/Working_Chart/Transparency.GoToExerciseHome.GoHome_M5.ST4_Abs_ref_start_immediatly_M5/receive_PDO1_m1 ==
  controlword : Inport
  CAN Write : speedgoatlib_IO614/CAN/CAN Write  id=1  sampleTime=-1  portSelection=4  messageType=CAN  enaStatusPort=off  protl=IO614  ptIdx=3  isFDMod=0
  set_controlword : canmsglib/CAN Pack  MsgList=(none)  MsgName=CAN Msg  MsgIDType=Standard (11-bit identifier)  MsgIdentifier=hex2dec('203')  MsgLength=2  Remote=off  ApplyMinMax=off  BusOutput=off  SignalInfo={ 'controlword', '0', '16', 'LE', 'unsigned', 'Standard', '0', '1', '0', '-Inf', 'Inf' }
      settings: DataFormat=manually specified signals
  wires:
  controlword/1 -> set_controlword/1
  set_controlword/1 -> CAN Write/1

== system ExoskeletonControlModel/DataProcessing/Working_Chart/Transparency.GoToExerciseHome.GoHome_M6.ST1_set_PPM_M6/receive_PDO2_m1 ==
  mode : Inport
  Bus Selector : BusSelector  OutputSignals=mode_m1,interpolation_period_m1
  CAN Write : speedgoatlib_IO614/CAN/CAN Write  id=1  sampleTime=-1  portSelection=4  messageType=CAN  enaStatusPort=off  protl=IO614  ptIdx=3  isFDMod=0
  set_mode : canmsglib/CAN Pack  MsgList=(none)  MsgName=CAN Msg  MsgIDType=Standard (11-bit identifier)  MsgIdentifier=hex2dec('304')  MsgLength=2  Remote=off  ApplyMinMax=off  BusOutput=off  SignalInfo={ 'mode', '0', '8', 'LE', 'unsigned', 'Standard', '0', '1', '0', '-Inf', 'Inf'; 'interpolation time period', '8', '8', 'LE', 'unsigned', 'Standard', '0', '1', '0', '-Inf', 'Inf' }
      settings: DataFormat=manually specified signals
  wires:
  set_mode/1 -> CAN Write/1
  mode/1 -> Bus Selector/1
  Bus Selector/1 -> set_mode/1  "<mode_m1>"
  Bus Selector/2 -> set_mode/2  "<interpolation_period_m1>"

== system ExoskeletonControlModel/DataProcessing/Working_Chart/Transparency.GoToExerciseHome.GoHome_M6.ST2_Switch_on_Enable_M6/receive_PDO1_m1 ==
  controlword : Inport
  CAN Write : speedgoatlib_IO614/CAN/CAN Write  id=1  sampleTime=-1  portSelection=4  messageType=CAN  enaStatusPort=off  protl=IO614  ptIdx=3  isFDMod=0
  set_controlword : canmsglib/CAN Pack  MsgList=(none)  MsgName=CAN Msg  MsgIDType=Standard (11-bit identifier)  MsgIdentifier=hex2dec('204')  MsgLength=2  Remote=off  ApplyMinMax=off  BusOutput=off  SignalInfo={ 'controlword', '0', '16', 'LE', 'unsigned', 'Standard', '0', '1', '0', '-Inf', 'Inf' }
      settings: DataFormat=manually specified signals
  wires:
  controlword/1 -> set_controlword/1
  set_controlword/1 -> CAN Write/1

== system ExoskeletonControlModel/DataProcessing/Working_Chart/Transparency.GoToExerciseHome.GoHome_M6.ST3_send_target_pos_M6/receive_PDO3_m1 ==
  target_pos : Inport
  CAN Write : speedgoatlib_IO614/CAN/CAN Write  id=1  sampleTime=-1  portSelection=4  messageType=CAN  enaStatusPort=off  protl=IO614  ptIdx=3  isFDMod=0
  set_position : canmsglib/CAN Pack  MsgList=(none)  MsgName=CAN Msg  MsgIDType=Standard (11-bit identifier)  MsgIdentifier=hex2dec('404')  MsgLength=4  Remote=off  ApplyMinMax=off  BusOutput=off  SignalInfo={ 'target position', '0', '32', 'LE', 'signed', 'Standard', '0', '1', '0', '-Inf', 'Inf' }
      settings: DataFormat=manually specified signals
  wires:
  target_pos/1 -> set_position/1
  set_position/1 -> CAN Write/1

== system ExoskeletonControlModel/DataProcessing/Working_Chart/Transparency.GoToExerciseHome.GoHome_M6.ST4_Abs_ref_start_immediatly_M6/receive_PDO1_m1 ==
  controlword : Inport
  CAN Write : speedgoatlib_IO614/CAN/CAN Write  id=1  sampleTime=-1  portSelection=4  messageType=CAN  enaStatusPort=off  protl=IO614  ptIdx=3  isFDMod=0
  set_controlword : canmsglib/CAN Pack  MsgList=(none)  MsgName=CAN Msg  MsgIDType=Standard (11-bit identifier)  MsgIdentifier=hex2dec('204')  MsgLength=2  Remote=off  ApplyMinMax=off  BusOutput=off  SignalInfo={ 'controlword', '0', '16', 'LE', 'unsigned', 'Standard', '0', '1', '0', '-Inf', 'Inf' }
      settings: DataFormat=manually specified signals
  wires:
  controlword/1 -> set_controlword/1
  set_controlword/1 -> CAN Write/1

== system ExoskeletonControlModel/DataProcessing/Working_Chart/Transparency.ImpedanceMode.ShoulderFlexion.ST1_set_CSP_M3/receive_PDO2_m1 ==
  mode : Inport
  Bus Selector : BusSelector  OutputSignals=mode_m1,interpolation_period_m1
  CAN Write : speedgoatlib_IO614/CAN/CAN Write  id=1  sampleTime=-1  portSelection=4  messageType=CAN  enaStatusPort=off  protl=IO614  ptIdx=3  isFDMod=0
  set_mode : canmsglib/CAN Pack  MsgList=(none)  MsgName=CAN Msg  MsgIDType=Standard (11-bit identifier)  MsgIdentifier=hex2dec('301')  MsgLength=2  Remote=off  ApplyMinMax=off  BusOutput=off  SignalInfo={ 'mode', '0', '8', 'LE', 'unsigned', 'Standard', '0', '1', '0', '-Inf', 'Inf'; 'interpolation time period', '8', '8', 'LE', 'unsigned', 'Standard', '0', '1', '0', '-Inf', 'Inf' }
      settings: DataFormat=manually specified signals
  wires:
  set_mode/1 -> CAN Write/1
  mode/1 -> Bus Selector/1
  Bus Selector/1 -> set_mode/1  "<mode_m1>"
  Bus Selector/2 -> set_mode/2  "<interpolation_period_m1>"

== system ExoskeletonControlModel/DataProcessing/Working_Chart/Transparency.ImpedanceMode.ShoulderFlexion.ST1_set_CSP_M4/receive_PDO2_m1 ==
  mode : Inport
  Bus Selector : BusSelector  OutputSignals=mode_m1,interpolation_period_m1
  CAN Write : speedgoatlib_IO614/CAN/CAN Write  id=1  sampleTime=-1  portSelection=4  messageType=CAN  enaStatusPort=off  protl=IO614  ptIdx=3  isFDMod=0
  set_mode : canmsglib/CAN Pack  MsgList=(none)  MsgName=CAN Msg  MsgIDType=Standard (11-bit identifier)  MsgIdentifier=hex2dec('302')  MsgLength=2  Remote=off  ApplyMinMax=off  BusOutput=off  SignalInfo={ 'mode', '0', '8', 'LE', 'unsigned', 'Standard', '0', '1', '0', '-Inf', 'Inf'; 'interpolation time period', '8', '8', 'LE', 'unsigned', 'Standard', '0', '1', '0', '-Inf', 'Inf' }
      settings: DataFormat=manually specified signals
  wires:
  set_mode/1 -> CAN Write/1
  mode/1 -> Bus Selector/1
  Bus Selector/1 -> set_mode/1  "<mode_m1>"
  Bus Selector/2 -> set_mode/2  "<interpolation_period_m1>"

== system ExoskeletonControlModel/DataProcessing/Working_Chart/Transparency.ImpedanceMode.ShoulderFlexion.ST1_set_CSP_M6/receive_PDO2_m1 ==
  mode : Inport
  Bus Selector : BusSelector  OutputSignals=mode_m1,interpolation_period_m1
  CAN Write : speedgoatlib_IO614/CAN/CAN Write  id=1  sampleTime=-1  portSelection=4  messageType=CAN  enaStatusPort=off  protl=IO614  ptIdx=3  isFDMod=0
  set_mode : canmsglib/CAN Pack  MsgList=(none)  MsgName=CAN Msg  MsgIDType=Standard (11-bit identifier)  MsgIdentifier=hex2dec('304')  MsgLength=2  Remote=off  ApplyMinMax=off  BusOutput=off  SignalInfo={ 'mode', '0', '8', 'LE', 'unsigned', 'Standard', '0', '1', '0', '-Inf', 'Inf'; 'interpolation time period', '8', '8', 'LE', 'unsigned', 'Standard', '0', '1', '0', '-Inf', 'Inf' }
      settings: DataFormat=manually specified signals
  wires:
  set_mode/1 -> CAN Write/1
  mode/1 -> Bus Selector/1
  Bus Selector/1 -> set_mode/1  "<mode_m1>"
  Bus Selector/2 -> set_mode/2  "<interpolation_period_m1>"

== system ExoskeletonControlModel/DataProcessing/Working_Chart/Transparency.SET_MODE.ST1_set_CSP_M2/receive_PDO2_m1 ==
  mode : Inport
  Bus Selector : BusSelector  OutputSignals=mode_m1,interpolation_period_m1
  CAN Write : speedgoatlib_IO614/CAN/CAN Write  id=1  sampleTime=-1  portSelection=3  messageType=CAN  enaStatusPort=off  protl=IO614  ptIdx=2  isFDMod=0
  set_mode : canmsglib/CAN Pack  MsgList=(none)  MsgName=CAN Msg  MsgIDType=Standard (11-bit identifier)  MsgIdentifier=hex2dec('302')  MsgLength=2  Remote=off  ApplyMinMax=off  BusOutput=off  SignalInfo={ 'mode', '0', '8', 'LE', 'unsigned', 'Standard', '0', '1', '0', '-Inf', 'Inf'; 'interpolation time period', '8', '8', 'LE', 'unsigned', 'Standard', '0', '1', '0', '-Inf', 'Inf' }
      settings: DataFormat=manually specified signals
  wires:
  set_mode/1 -> CAN Write/1
  mode/1 -> Bus Selector/1
  Bus Selector/1 -> set_mode/1  "<mode_m1>"
  Bus Selector/2 -> set_mode/2  "<interpolation_period_m1>"

== system ExoskeletonControlModel/DataProcessing/Working_Chart/Transparency.SET_MODE.ST1_set_CST_M1/receive_PDO2_m1 ==
  mode : Inport
  Bus Selector : BusSelector  OutputSignals=mode_m1,interpolation_period_m1
  CAN Write : speedgoatlib_IO614/CAN/CAN Write  id=1  sampleTime=-1  portSelection=3  messageType=CAN  enaStatusPort=off  protl=IO614  ptIdx=2  isFDMod=0
  set_mode : canmsglib/CAN Pack  MsgList=(none)  MsgName=CAN Msg  MsgIDType=Standard (11-bit identifier)  MsgIdentifier=hex2dec('301')  MsgLength=2  Remote=off  ApplyMinMax=off  BusOutput=off  SignalInfo={ 'mode', '0', '8', 'LE', 'unsigned', 'Standard', '0', '1', '0', '-Inf', 'Inf'; 'interpolation time period', '8', '8', 'LE', 'unsigned', 'Standard', '0', '1', '0', '-Inf', 'Inf' }
      settings: DataFormat=manually specified signals
  wires:
  set_mode/1 -> CAN Write/1
  mode/1 -> Bus Selector/1
  Bus Selector/1 -> set_mode/1  "<mode_m1>"
  Bus Selector/2 -> set_mode/2  "<interpolation_period_m1>"

== system ExoskeletonControlModel/DataProcessing/Working_Chart/Transparency.SET_MODE.ST1_set_CST_M3/receive_PDO2_m1 ==
  mode : Inport
  Bus Selector : BusSelector  OutputSignals=mode_m1,interpolation_period_m1
  CAN Write : speedgoatlib_IO614/CAN/CAN Write  id=1  sampleTime=-1  portSelection=4  messageType=CAN  enaStatusPort=off  protl=IO614  ptIdx=3  isFDMod=0
  set_mode : canmsglib/CAN Pack  MsgList=(none)  MsgName=CAN Msg  MsgIDType=Standard (11-bit identifier)  MsgIdentifier=hex2dec('301')  MsgLength=2  Remote=off  ApplyMinMax=off  BusOutput=off  SignalInfo={ 'mode', '0', '8', 'LE', 'unsigned', 'Standard', '0', '1', '0', '-Inf', 'Inf'; 'interpolation time period', '8', '8', 'LE', 'unsigned', 'Standard', '0', '1', '0', '-Inf', 'Inf' }
      settings: DataFormat=manually specified signals
  wires:
  set_mode/1 -> CAN Write/1
  mode/1 -> Bus Selector/1
  Bus Selector/1 -> set_mode/1  "<mode_m1>"
  Bus Selector/2 -> set_mode/2  "<interpolation_period_m1>"

== system ExoskeletonControlModel/DataProcessing/Working_Chart/Transparency.SET_MODE.ST1_set_CST_M4/receive_PDO2_m1 ==
  mode : Inport
  Bus Selector : BusSelector  OutputSignals=mode_m1,interpolation_period_m1
  CAN Write : speedgoatlib_IO614/CAN/CAN Write  id=1  sampleTime=-1  portSelection=4  messageType=CAN  enaStatusPort=off  protl=IO614  ptIdx=3  isFDMod=0
  set_mode : canmsglib/CAN Pack  MsgList=(none)  MsgName=CAN Msg  MsgIDType=Standard (11-bit identifier)  MsgIdentifier=hex2dec('302')  MsgLength=2  Remote=off  ApplyMinMax=off  BusOutput=off  SignalInfo={ 'mode', '0', '8', 'LE', 'unsigned', 'Standard', '0', '1', '0', '-Inf', 'Inf'; 'interpolation time period', '8', '8', 'LE', 'unsigned', 'Standard', '0', '1', '0', '-Inf', 'Inf' }
      settings: DataFormat=manually specified signals
  wires:
  set_mode/1 -> CAN Write/1
  mode/1 -> Bus Selector/1
  Bus Selector/1 -> set_mode/1  "<mode_m1>"
  Bus Selector/2 -> set_mode/2  "<interpolation_period_m1>"

== system ExoskeletonControlModel/DataProcessing/Working_Chart/Transparency.SET_MODE.ST1_set_CST_M5/receive_PDO2_m1 ==
  mode : Inport
  Bus Selector : BusSelector  OutputSignals=mode_m1,interpolation_period_m1
  CAN Write : speedgoatlib_IO614/CAN/CAN Write  id=1  sampleTime=-1  portSelection=4  messageType=CAN  enaStatusPort=off  protl=IO614  ptIdx=3  isFDMod=0
  set_mode : canmsglib/CAN Pack  MsgList=(none)  MsgName=CAN Msg  MsgIDType=Standard (11-bit identifier)  MsgIdentifier=hex2dec('303')  MsgLength=2  Remote=off  ApplyMinMax=off  BusOutput=off  SignalInfo={ 'mode', '0', '8', 'LE', 'unsigned', 'Standard', '0', '1', '0', '-Inf', 'Inf'; 'interpolation time period', '8', '8', 'LE', 'unsigned', 'Standard', '0', '1', '0', '-Inf', 'Inf' }
      settings: DataFormat=manually specified signals
  wires:
  set_mode/1 -> CAN Write/1
  mode/1 -> Bus Selector/1
  Bus Selector/1 -> set_mode/1  "<mode_m1>"
  Bus Selector/2 -> set_mode/2  "<interpolation_period_m1>"
